simulink model "SguanTest"  (R2025a)
settings: Solver=FixedStepAuto  StartTime=0.0  StopTime=5  FixedStep=0.001  MaxStep=0.05  RelTol=1e-3
InitFcn:
  | Wn = 10;
  | zeta = 0.707;
  | 
  | Wd = Wn*sqrt(1-zeta^2);
  | tr = (pi - atan(sqrt(1-zeta^2)/zeta))/Wd;
  | tp = pi/Wd;
  | Mp = exp(1)^(-zeta*pi/sqrt(1-zeta^2));
  | ts002 = 4/(zeta*Wn);
  | ts005 = 3/(zeta*Wn);
  | N = ts002/(2*pi/Wd);
undefined symbols (not defined in the file): dspblkCoreblockFVToolHelper, gcbh
settings Model: Creator=星必尘Sguan  LastModifiedBy=星必尘Sguan
settings RTWCC: GenCodeOnly=on

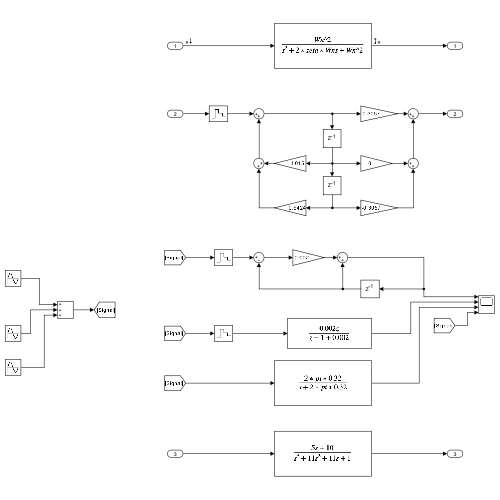
[thumbnail: Simulink's stored preview of the top-level diagram]
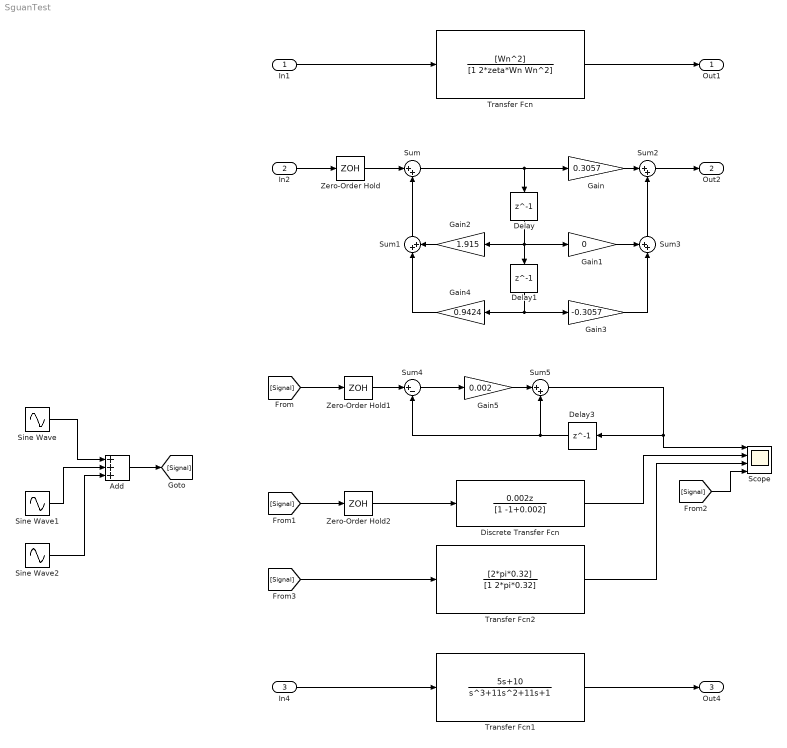
== system SguanTest ==
  In1 : Inport
  In2 : Inport  Port=2
  In4 : Inport  Port=3
  Add : Sum  Inputs=+++
  Delay : Delay  DelayLength=1
  Delay1 : Delay  DelayLength=1
  Delay3 : Delay  DelayLength=1
  Discrete Transfer Fcn : DiscreteTransferFcn  LoadFcn=dspblkCoreblockFVToolHelper(gcbh,'load');  Numerator=[0.002 0]  Denominator=[1 -1+0.002]
      settings: CopyFcn=dspblkCoreblockFVToolHelper(gcbh,'copy');  DeleteFcn=dspblkCoreblockFVToolHelper(gcbh,'close');  ModelCloseFcn=dspblkCoreblockFVToolHelper(gcbh,'close');  PreSaveFcn=dspblkCoreblockFVToolHelper(gcbh,'presave');  PostSaveFcn=dspblkCoreblockFVToolHelper(gcbh,'postsave');  CloseFcn=dspblkCoreblockFVToolHelper(gcbh,'close');
  Gain : Gain  Gain=0.3057
  Gain1 : Gain  Gain=0
  Gain2 : Gain  Gain=1.915
  Gain3 : Gain  Gain=-0.3057
  Gain4 : Gain  Gain=0.9424
  Gain5 : Gain  Gain=0.002
  Scope : Scope  NumInputPorts=4
      settings: ActiveDisplayYMinimum=-331.12804809687742  ActiveDisplayYMaximum=303.83689548833263
  Sine Wave : Sin  Amplitude=200  SampleTime=0
  Sine Wave1 : Sin  Amplitude=10  Frequency=50  SampleTime=0
  Sine Wave2 : Sin  Amplitude=3  Frequency=200  SampleTime=0
  Sum{,1..2,5} (4 alike) : Sum  Inputs=|++
  Sum3 : Sum  Inputs=++|
  Sum4 : Sum  Inputs=|+-
  Transfer Fcn : TransferFcn  Numerator=[Wn^2]  Denominator=[1 2*zeta*Wn Wn^2]
  Transfer Fcn1 : TransferFcn  Numerator=[5 10]  Denominator=[1 11 11 1]
  Transfer Fcn2 : TransferFcn  Numerator=[2*pi*0.32]  Denominator=[1 2*pi*0.32]
  Zero-Order Hold : ZeroOrderHold  SampleTime=0.001
  Zero-Order Hold1 : ZeroOrderHold  SampleTime=0.001
  Zero-Order Hold2 : ZeroOrderHold  SampleTime=0.001
  Out1 : Outport
  Out2 : Outport  Port=2
  Out4 : Outport  Port=3
  wires:
  Transfer Fcn/1 -> Out1/1
  In1/1 -> Transfer Fcn/1
  In2/1 -> Zero-Order Hold/1
  Zero-Order Hold/1 -> Sum/1
  Delay/1 -> Gain2/1, Gain1/1, Delay1/1
  Sum/1 -> Delay/1, Gain/1
  Sum1/1 -> Sum/2
  Gain2/1 -> Sum1/2
  Gain4/1 -> Sum1/1
  Delay1/1 -> Gain4/1, Gain3/1
  Gain1/1 -> Sum3/1
  Gain3/1 -> Sum3/2
  Sum3/1 -> Sum2/2
  Sum2/1 -> Out2/1
  Gain/1 -> Sum2/1
  Sum4/1 -> Gain5/1
  Delay3/1 -> Sum5/2, Sum4/2
  Gain5/1 -> Sum5/1
  Sum5/1 -> Delay3/1, Scope/1
  Zero-Order Hold1/1 -> Sum4/1
  In4/1 -> Transfer Fcn1/1
  Transfer Fcn1/1 -> Out4/1
  Zero-Order Hold2/1 -> Discrete Transfer Fcn/1
  Sine Wave/1 -> Add/1
  Sine Wave1/1 -> Add/2
  Sine Wave2/1 -> Add/3
  Add/1 -> [Signal]
  [Signal] -> Zero-Order Hold1/1
  [Signal] -> Zero-Order Hold2/1
  Discrete Transfer Fcn/1 -> Scope/2
  [Signal] -> Scope/4
  Transfer Fcn2/1 -> Scope/3
  [Signal] -> Transfer Fcn2/1
